simulink model "carsim"  (R2022b)
settings: Solver=FixedStepDiscrete  StartTime=0.0  StopTime=30  FixedStep=0.0005  RelTol=1e-3
values from neighbouring files (symbols this model uses):
  kappar = kxys    [path_design.m]
  thetar = yaw    [path_design.m]
  xr = px_spline'    [path_design.m]
  yr = py_spline'    [path_design.m]
libraries: Solver_SF x1
settings Model: Creator=Administrator  LastModifiedBy=Administrator
settings DataIOCC: ReturnWorkspaceOutputs=off

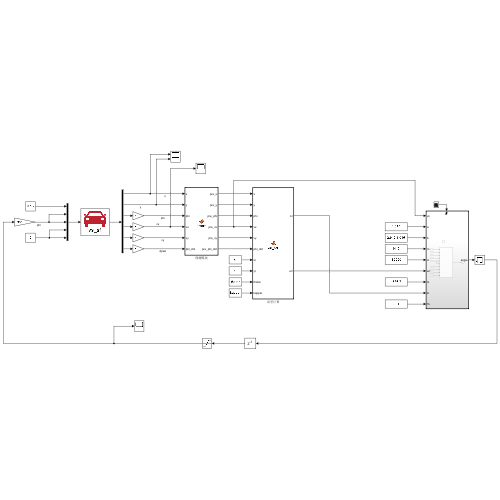
[thumbnail: Simulink's stored preview of the top-level diagram]
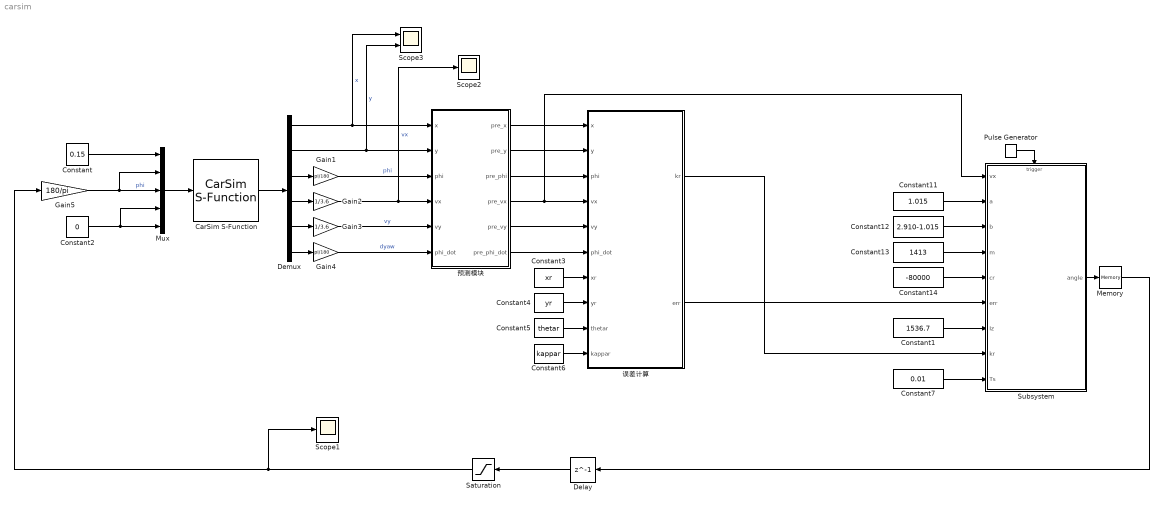
== system carsim ==
  CarSim S-Function : Solver_SF/CarSim S-Function  Priority=1  SIMFILE=E:\CarSim2020.0_Data\simfile.sim  Run_RTs=off  vs_state_ind=Run  StopMode_ind=Vehicle Model
  Constant : Constant  Value=0.15
  Constant1 : Constant  Value=1536.7
  Constant11 : Constant  Value=1.015
  Constant12 : Constant  Value=2.910-1.015
  Constant13 : Constant  Value=1413
  Constant14 : Constant  Value=-80000
  Constant2 : Constant  Value=0
  Constant3 : Constant  Value=xr
  Constant4 : Constant  Value=yr
  Constant5 : Constant  Value=thetar
  Constant6 : Constant  Value=kappar
  Constant7 : Constant  Value=0.01
  Delay : Delay  DelayLength=1  InitialCondition=0
  Demux : Demux  Outputs=6
  Gain1 : Gain  Gain=pi/180
  Gain2 : Gain  Gain=1/3.6
  Gain3 : Gain  Gain=1/3.6
  Gain4 : Gain  Gain=pi/180
  Gain5 : Gain  Gain=180/pi
  Memory : Memory  InheritSampleTime=on  LinearizeAsDelay=on
  Mux : Mux  Inputs=5
  Pulse Generator : DiscretePulseGenerator  PulseType=Time based  Period=0.01  PulseWidth=5
  Saturation : Saturate  UpperLimit=1.2  LowerLimit=-1.2
  Scope1 : Scope
  Scope2 : Scope
  Scope3 : Scope  NumInputPorts=2
  Subsystem : Subsystem
  误差计算 : MATLAB Function  TreatAsAtomicUnit=on
  预测模块 : MATLAB Function  TreatAsAtomicUnit=on
  wires:
  CarSim S-Function/1 -> Demux/1
  Mux/1 -> CarSim S-Function/1
  Constant/1 -> Mux/1
  Demux/4 -> Gain2/1
  Demux/3 -> Gain1/1
  Demux/5 -> Gain3/1
  Demux/6 -> Gain4/1
  Demux/1 -> 预测模块/1(x), Scope3/1  "x"
  Demux/2 -> 预测模块/2(y), Scope3/2  "y"
  Gain1/1 -> 预测模块/3(phi)  "phi"
  Gain2/1 -> 预测模块/4(vx), Scope2/1  "vx"
  Gain3/1 -> 预测模块/5(vy)  "vy"
  Gain4/1 -> 预测模块/6(phi_dot)  "dyaw"
  预测模块/1(pre_x) -> 误差计算/1(x)
  预测模块/2(pre_y) -> 误差计算/2(y)
  预测模块/3(pre_phi) -> 误差计算/3(phi)
  预测模块/4(pre_vx) -> 误差计算/4(vx), Subsystem/1(vx)
  预测模块/6(pre_phi_dot) -> 误差计算/6(phi_dot)
  Constant3/1 -> 误差计算/7(xr)
  预测模块/5(pre_vy) -> 误差计算/5(vy)
  Constant5/1 -> 误差计算/9(thetar)
  Constant4/1 -> 误差计算/8(yr)
  Constant6/1 -> 误差计算/10(kappar)
  Constant11/1 -> Subsystem/2(a)
  Constant12/1 -> Subsystem/3(b)
  Constant13/1 -> Subsystem/4(m)
  Constant14/1 -> Subsystem/5(cr)
  误差计算/1(kr) -> Subsystem/8(kr)
  Memory/1 -> Delay/1
  Delay/1 -> Saturation/1
  Saturation/1 -> Scope1/1, Gain5/1
  Gain5/1 -> Mux/3, Mux/2  "phi"
  Constant2/1 -> Mux/4, Mux/5
  误差计算/2(err) -> Subsystem/6(err)
  Constant1/1 -> Subsystem/7(Iz)
  Constant7/1 -> Subsystem/9(Ts)
  Subsystem/1(angle) -> Memory/1
  Pulse Generator/1 -> Subsystem/Trigger

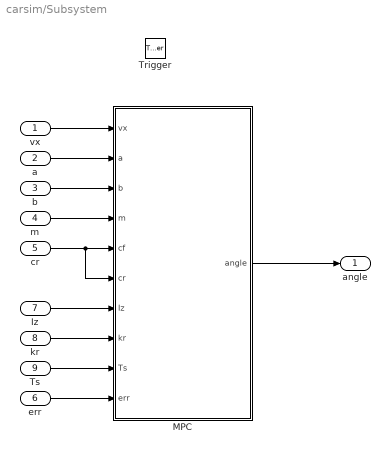
== system carsim/Subsystem ==
  vx : Inport
  a : Inport  Port=2
  b : Inport  Port=3
  m : Inport  Port=4
  cr : Inport  Port=5
  err : Inport  Port=6
  Iz : Inport  Port=7
  kr : Inport  Port=8
  Ts : Inport  Port=9
  Trigger : TriggerPort  VariantControl=(inherit)  PortDimensions=1
  MPC : MATLAB Function  TreatAsAtomicUnit=on
  angle : Outport
  wires:
  cr/1 -> MPC/6(cr), MPC/5(cf)
  a/1 -> MPC/2(a)
  Ts/1 -> MPC/9(Ts)
  m/1 -> MPC/4(m)
  Iz/1 -> MPC/7(Iz)
  b/1 -> MPC/3(b)
  vx/1 -> MPC/1(vx)
  MPC/1(angle) -> angle/1
  err/1 -> MPC/10(err)
  kr/1 -> MPC/8(kr)

== matlab function carsim/误差计算 ==
  data: x input; kr output; y input; phi input; vx input; vy input; phi_dot input; xr input; yr input; thetar input; kappar input; err output
function [kr,err] = err_cal(x,y,phi,vx,vy,phi_dot,xr,yr,thetar,kappar)
    n=length(xr);
    d_min=(x-xr(1))^2+(y-yr(1))^2;
    min=1;
    for i=1:n
        d=(x-xr(i))^2+(y-yr(i))^2;
        if d<d_min
            d_min=d;
            min=i;
        end
    end
    dmin=min;
    tor=[cos(thetar(dmin));sin(thetar(dmin))];
    nor=[-sin(thetar(dmin));cos(thetar(dmin))];
    d_err=[x-xr(dmin);y-yr(dmin)];
    ed=nor'*d_err;
    es=tor'*d_err;
    %projection_point_thetar=thetar(dmin);%apollo
    projection_point_thetar=thetar(dmin)+kappar(dmin)*es;
    ed_dot=vy*cos(phi-projection_point_thetar)+vx*sin(phi-projection_point_thetar);
    %%%%%%%%%
    ephi=sin(phi-projection_point_thetar);%去除2pi差距的影响
    %%%%%%%%%
    s_dot=vx*cos(phi-projection_point_thetar)-vy*sin(phi-projection_point_thetar);
    s_dot=s_dot/(1-kappar(dmin)*ed);
    ephi_dot=phi_dot-kappar(dmin)*s_dot;
    kr=kappar(dmin);
    err=[ed;ed_dot;ephi;ephi_dot];
    

end

== matlab function carsim/预测模块 ==
  data: x input; pre_x output; y input; phi input; vx input; vy input; phi_dot input; pre_y output; pre_phi output; pre_vx output; pre_vy output; pre_phi_dot output
function [pre_x,pre_y,pre_phi,pre_vx,pre_vy,pre_phi_dot] = predict(x,y,phi,vx,vy,phi_dot)
% 预测函数（模拟司机）
% Detailed explanation goes here

ts=0.1;
pre_x=x+vx*ts*cos(phi)-vy*ts*sin(phi);
pre_y=y+vy*ts*cos(phi)+vx*ts*sin(phi);
pre_phi=phi+phi_dot*ts;
pre_vx=vx;
pre_vy=vy;
pre_phi_dot=phi_dot;

end

== matlab function carsim/Subsystem/MPC ==
  data: vx input; angle output; a input; b input; m input; cf input; cr input; Iz input; kr input; Ts input; err input
function angle = mpc(vx,a,b,m,cf,cr,Iz,kr, Ts,err)

%MPC参数矩阵
% 定义Q矩阵，n x n 矩阵
Q=diag([100 5 50 10]);
% 定义F矩阵，n x n 矩阵
F=diag([100 5 50 10]);
% 定义R矩阵，p x p 矩阵
R=30;

%预测步数
N=15;

[A,B] = getAB(vx,a,b,m,cf,cr,Iz,Ts);
[E,H] = MPC_Matrices(A,B,Q,R,F,N);%计算下一个E H
angle = Prediction(err,E,H,N,1);

% MPC暂时没找到前馈补偿的方法
% 最小二乘前馈补偿
% if(vx>0.01) 
%     C = [0 (a*cf-b*cr)/m/vx-vx 0 (a*a*cf+b*b*cr)/Iz/vx]';
%     angle = angle - (B'*B)^-1 * B' * C *kr*vx;
% end
